simulink model "ACC_Model_by_GL"  (R2023a)
settings: Solver=ode1  StartTime=0.0  StopTime=60  FixedStep=0.001  RelTol=1e-3
settings Model: Creator=guanyunliu  LastModifiedBy=guanyunliu
settings DebuggingCC: UnconnectedInputMsg=warning  UnconnectedOutputMsg=warning  UnconnectedLineMsg=warning
settings ModelReferenceCC: EnableRefExpFcnMdlSchedulingChecks=on
settings RTWCC: DLArmComputeVersion=19.05

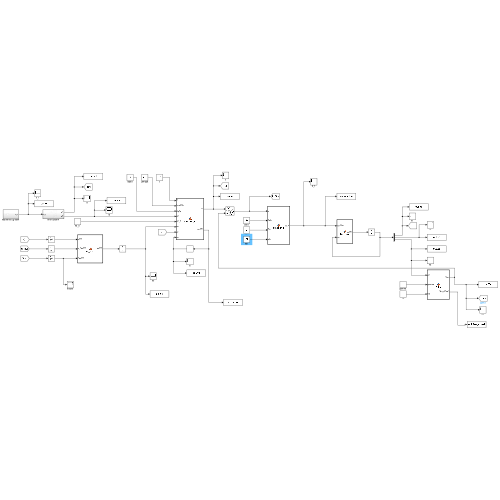
[thumbnail: Simulink's stored preview of the top-level diagram]
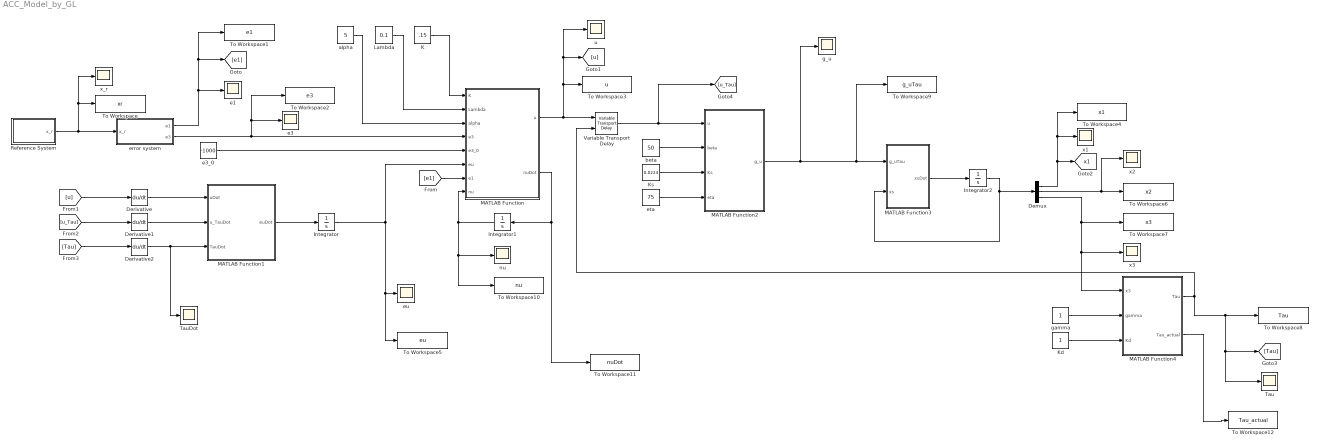
== system ACC_Model_by_GL ==
  Demux : Demux  Outputs=3
  Derivative : Derivative
  Derivative1 : Derivative
  Derivative2 : Derivative
  Integrator : Integrator
  Integrator1 : Integrator
  Integrator2 : Integrator  InitialCondition=[500;50;5]
  K : Constant  Value=.15
  Kd : Constant
  Ks : Constant  Value=0.0224
  Lambda : Constant  Value=0.1
  MATLAB Function : MATLAB Function  TreatAsAtomicUnit=on
  MATLAB Function1 : MATLAB Function  TreatAsAtomicUnit=on
  MATLAB Function2 : MATLAB Function  TreatAsAtomicUnit=on
  MATLAB Function3 : MATLAB Function  TreatAsAtomicUnit=on
  MATLAB Function4 : MATLAB Function  TreatAsAtomicUnit=on
  Reference System : Subsystem
  Tau : Scope
  TauDot : Scope
  To Workspace : ToWorkspace  VariableName=xr  SaveFormat=Timeseries  SampleTime=-1
  To Workspace1 : ToWorkspace  VariableName=e1  SaveFormat=Timeseries  SampleTime=-1
  To Workspace10 : ToWorkspace  VariableName=nu  SaveFormat=Timeseries  SampleTime=-1
  To Workspace11 : ToWorkspace  VariableName=nuDot  SaveFormat=Timeseries  SampleTime=-1
  To Workspace12 : ToWorkspace  VariableName=Tau_actual  SaveFormat=Timeseries  SampleTime=-1
  To Workspace2 : ToWorkspace  VariableName=e3  SaveFormat=Timeseries  SampleTime=-1
  To Workspace3 : ToWorkspace  VariableName=u  SaveFormat=Timeseries  SampleTime=-1
  To Workspace4 : ToWorkspace  VariableName=x1  SaveFormat=Timeseries  SampleTime=-1
  To Workspace5 : ToWorkspace  VariableName=eu  SaveFormat=Timeseries  SampleTime=-1
  To Workspace6 : ToWorkspace  VariableName=x2  SaveFormat=Timeseries  SampleTime=-1
  To Workspace7 : ToWorkspace  VariableName=x3  SaveFormat=Timeseries  SampleTime=-1
  To Workspace8 : ToWorkspace  VariableName=Tau  SaveFormat=Timeseries  SampleTime=-1
  To Workspace9 : ToWorkspace  VariableName=g_uTau  SaveFormat=Timeseries  SampleTime=-1
  Variable Transport Delay : VariableTransportDelay  VariableDelayType=Variable transport delay  MaximumDelay=10  MaximumPoints=10240
  alpha : Constant  Value=5
  beta : Constant  Value=50
  e1 : Scope
  e3 : Scope
  e3_0 : Constant  Value=-1000
  error system : Subsystem
  eta : Constant  Value=75
  eu : Scope
  g_u : Scope
  gamma : Constant
  nu : Scope
  u : Scope
  x1 : Scope
  x2 : Scope
  x3 : Scope
  x_r : Scope
  tag scope: x1=global
  wires:
  Reference System/1(x_r) -> To Workspace/1, x_r/1, error system/1(x_r)
  error system/1(e1) -> To Workspace1/1, [e1], e1/1
  error system/2(e3) -> MATLAB Function/4(e3), To Workspace2/1, e3/1
  alpha/1 -> MATLAB Function/3(alpha)
  K/1 -> MATLAB Function/1(K)
  Lambda/1 -> MATLAB Function/2(Lambda)
  e3_0/1 -> MATLAB Function/5(e3_0)
  [e1] -> MATLAB Function/7(e1)
  MATLAB Function/2(nuDot) -> To Workspace11/1, Integrator1/1
  Integrator1/1 -> To Workspace10/1, nu/1, MATLAB Function/8(nu)
  [u] -> Derivative/1
  Derivative/1 -> MATLAB Function1/1(uDot)
  [u_Tau] -> Derivative1/1
  Derivative1/1 -> MATLAB Function1/2(u_TauDot)
  Derivative2/1 -> TauDot/1, MATLAB Function1/3(TauDot)
  MATLAB Function1/1(euDot) -> Integrator/1
  Integrator/1 -> To Workspace5/1, eu/1, MATLAB Function/6(eu)
  MATLAB Function/1(u) -> [u], u/1, To Workspace3/1, Variable Transport Delay/1
  beta/1 -> MATLAB Function2/2(beta)
  Ks/1 -> MATLAB Function2/3(Ks)
  eta/1 -> MATLAB Function2/4(eta)
  MATLAB Function2/1(g_u) -> g_u/1, To Workspace9/1, MATLAB Function3/1(g_uTau)
  MATLAB Function3/1(xsDot) -> Integrator2/1
  Integrator2/1 -> Demux/1, MATLAB Function3/2(xs)
  Demux/1 -> [x1], x1/1, To Workspace4/1
  Demux/2 -> x2/1, To Workspace6/1
  Demux/3 -> x3/1, MATLAB Function4/1(x3), To Workspace7/1
  gamma/1 -> MATLAB Function4/2(gamma)
  Kd/1 -> MATLAB Function4/3(Kd)
  MATLAB Function4/1(Tau) -> Tau/1, [Tau], To Workspace8/1, Variable Transport Delay/2
  [Tau] -> Derivative2/1
  Variable Transport Delay/1 -> [u_Tau], MATLAB Function2/1(u)
  MATLAB Function4/2(Tau_actual) -> To Workspace12/1

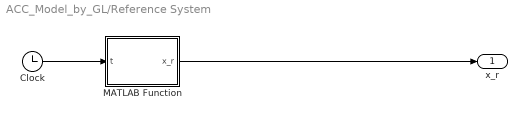
== system ACC_Model_by_GL/Reference System ==
  Clock : Clock
  MATLAB Function : MATLAB Function  TreatAsAtomicUnit=on
  x_r : Outport
  wires:
  Clock/1 -> MATLAB Function/1(t)
  MATLAB Function/1(x_r) -> x_r/1

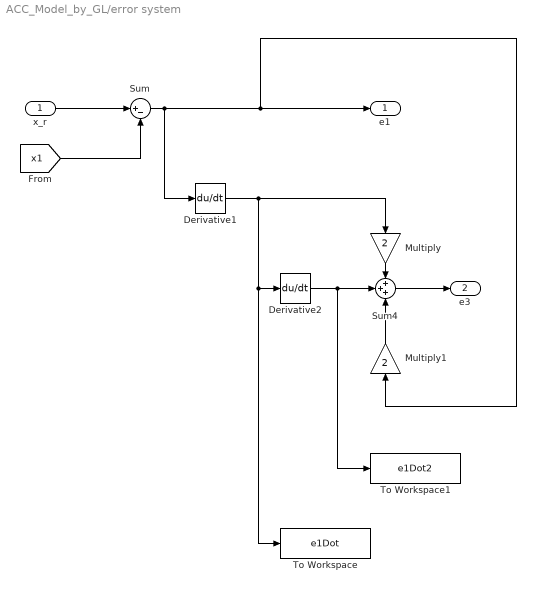
== system ACC_Model_by_GL/error system ==
  x_r : Inport
  Derivative1 : Derivative
  Derivative2 : Derivative
  Multiply : Gain  Gain=2
  Multiply1 : Gain  Gain=2
  Sum : Sum  Inputs=|+-
  Sum4 : Sum  Inputs=+++
  To Workspace : ToWorkspace  VariableName=e1Dot  SaveFormat=Timeseries  SampleTime=-1
  To Workspace1 : ToWorkspace  VariableName=e1Dot2  SaveFormat=Timeseries  SampleTime=-1
  e1 : Outport
  e3 : Outport  Port=2
  wires:
  x_r/1 -> Sum/1
  [x1] -> Sum/2
  Sum/1 -> Derivative1/1, e1/1, Multiply1/1
  Derivative2/1 -> To Workspace1/1, Sum4/2
  Multiply/1 -> Sum4/1
  Multiply1/1 -> Sum4/3
  Sum4/1 -> e3/1
  Derivative1/1 -> Multiply/1, To Workspace/1, Derivative2/1

== matlab function ACC_Model_by_GL/MATLAB Function1 ==
  data: uDot input; euDot output; u_TauDot input; TauDot input
function euDot = eu_error(uDot,u_TauDot, TauDot)

euDot = -uDot+(1-TauDot)*u_TauDot;

== matlab function ACC_Model_by_GL/MATLAB Function ==
  data: K input; u output; Lambda input; alpha input; e3 input; e3_0 input; eu input; e1 input; nu input; nuDot output
function [u, nuDot] = controller_u(K, Lambda, alpha, e3, e3_0, eu, e1, nu)
u = (sign(0.5 * (sign(e1) + 1))) * ...
    (K * (e3 - e3_0) + nu);
nuDot = K * (Lambda*e3+alpha*eu);
return

== matlab function ACC_Model_by_GL/MATLAB Function2 ==
  data: u input; g_u output; beta input; Ks input; eta input
function g_u = controller_g(u,beta, Ks, eta)

g_u = (beta/2)+((beta/2)*tanh(Ks/2*(u-eta)));

return

== matlab function ACC_Model_by_GL/MATLAB Function3 ==
  data: g_uTau input; xsDot output; xs input
function xsDot = Dynamics(g_uTau, xs)
% Parameters
d1 = 1.1311;
d2 = 1.1362;
d3 = 0.2727;

x1 = xs(1);
x2 = xs(2);
x3 = xs(3);

x1dot = -d1 * x1 + x2;
x2dot = -d2 * x2 + x3;
x3dot = -d3 * x3 + g_uTau;

xsDot = [x1dot; x2dot; x3dot];

== matlab function ACC_Model_by_GL/MATLAB Function4 ==
  data: x3 input; Tau output; gamma input; Kd input; Tau_actual output
function [Tau, Tau_actual]= Delay(x3, gamma, Kd)
% Tau=(4.48*(max(x3,.202)^(-0.323))) ; From Damon's code
% Tau = gamma * x3^(-Kd);
Tau = gamma * 5^(-Kd);
Tau_actual = gamma * x3^(-Kd);
return

== matlab function ACC_Model_by_GL/Reference System/MATLAB Function ==
  data: t input; x_r output
function x_r = fcn(t)

% x_r =(200*sin(.25*t)+300).*(1-exp(-t.^.5));

% x_r =(100*sin(.15*t)+300); 

% x_r=125*(tanh(0.15*t)^2);
x_r = 130 + 30*sin(0.17*t);
